simulink model "TwoTimeScale_Plant"  (R2023a)
settings: Solver=ode4  StartTime=0.0  StopTime=2  FixedStep=0.0005  RelTol=1e-3
settings Model: Creator=Fasih  LastModifiedBy=Fasih

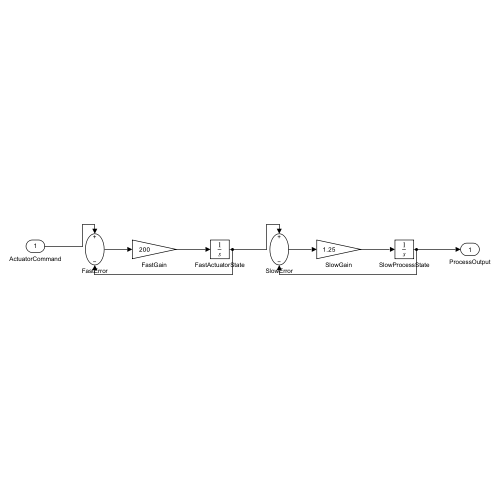
[thumbnail: Simulink's stored preview of the top-level diagram]
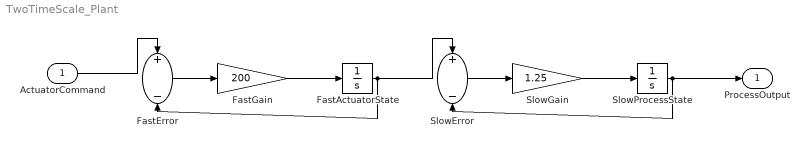
== system TwoTimeScale_Plant ==
  ActuatorCommand : Inport
  FastActuatorState : Integrator
  FastError : Sum  Inputs=+-
  FastGain : Gain  Gain=200
  SlowError : Sum  Inputs=+-
  SlowGain : Gain  Gain=1.25
  SlowProcessState : Integrator
  ProcessOutput : Outport
  wires:
  ActuatorCommand/1 -> FastError/1
  FastActuatorState/1 -> FastError/2, SlowError/1
  FastError/1 -> FastGain/1
  FastGain/1 -> FastActuatorState/1
  SlowProcessState/1 -> SlowError/2, ProcessOutput/1
  SlowError/1 -> SlowGain/1
  SlowGain/1 -> SlowProcessState/1
